simulink model "project"  (R2023b)
settings: Solver=VariableStepAuto  StartTime=0.0  StopTime=sim_time  RelTol=1e-3
undefined symbols (not defined in the file): b1, b2, F, k1, k2, m1, m2
settings Model: Creator=Henrique  LastModifiedBy=Henrique

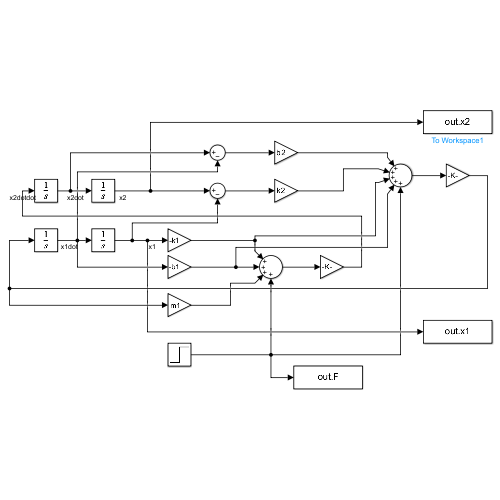
[thumbnail: Simulink's stored preview of the top-level diagram]
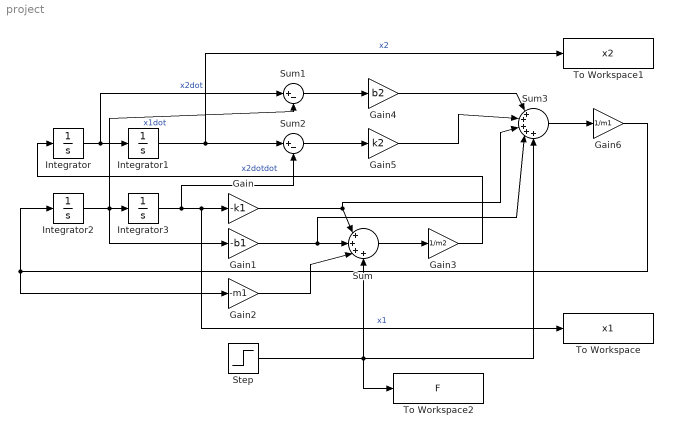
== system project ==
  Gain : Gain  Gain=-k1
  Gain1 : Gain  Gain=-b1
  Gain2 : Gain  Gain=-m1
  Gain3 : Gain  Gain=1/m2
  Gain4 : Gain  Gain=b2
  Gain5 : Gain  Gain=k2
  Gain6 : Gain  Gain=1/m1
  Integrator{,1..3} (4 alike) : Integrator
  Step : Step  After=F  SampleTime=0
  Sum : Sum  Inputs=|++++
  Sum1 : Sum  Inputs=|+-
  Sum2 : Sum  Inputs=|+-
  Sum3 : Sum  Inputs=|+++++
  To Workspace : ToWorkspace  VariableName=x1  SaveFormat=Timeseries  SampleTime=-1
  To Workspace1 : ToWorkspace  VariableName=x2  SaveFormat=Timeseries  SampleTime=-1
  To Workspace2 : ToWorkspace  VariableName=F  SaveFormat=Timeseries  SampleTime=-1
  wires:
  Gain3/1 -> Integrator/1  "x2dotdot"
  Integrator/1 -> Sum1/1, Integrator1/1  "x2dot"
  Integrator1/1 -> To Workspace1/1, Sum2/1  "x2"
  Integrator2/1 -> Sum1/2, Gain1/1, Integrator3/1  "x1dot"
  Integrator3/1 -> Sum2/2, To Workspace/1, Gain/1  "x1"
  Gain6/1 -> Integrator2/1, Gain2/1
  Gain/1 -> Sum/1, Sum3/3
  Gain1/1 -> Sum3/4, Sum/2
  Gain2/1 -> Sum/3
  Step/1 -> Sum3/5, To Workspace2/1, Sum/4
  Sum/1 -> Gain3/1
  Sum1/1 -> Gain4/1
  Sum2/1 -> Gain5/1
  Gain4/1 -> Sum3/1
  Gain5/1 -> Sum3/2
  Sum3/1 -> Gain6/1
